simulink model "MIL4L3_SW6_V1_20220211"  (R2018b)
settings: Solver=FixedStepAuto  StartTime=0.0  StopTime=inf  FixedStep=0.001  RelTol=1e-3
PreLoadFcn:
  | A0_MILtest;
undefined symbols (not defined in the file or in its folder): Clb_ICADirect_LaneDisp_StateFive, Clb_ICADirect_LaneDisp_StateFour, Clb_ICADirect_LaneDisp_StateOne, Clb_ICADirect_LaneDisp_StateThree, Clb_ICADirect_LaneDisp_StateTwo, Clb_ICADirect_LaneDisp_StateZero, Clb_ICADirect_LaneDispSW, Clb_ICADirect_TrnLghtsCom_Switch, Clb_ICADirect_TrnLghtsCom_Value, Clb_ICADirect_TrnLghtsCrtl_Inhb, IMAP_Clb_ACU_Driver_Belt, IMAP_Clb_ACU_Driver_Belt_Over, IMAP_Clb_ACU_Passenger_Belt, IMAP_Clb_ACU_Passenger_Belt_Over, IMAP_Clb_ACU_RearLeft_Belt, IMAP_Clb_ACU_RearLeft_Belt_Over, IMAP_Clb_ACU_RearMiddle_Belt, IMAP_Clb_ACU_RearMiddle_Belt_Over, IMAP_Clb_ACU_RearRight_Belt, IMAP_Clb_ACU_RearRight_Belt_Over, IMAP_Clb_AEB_Switch, IMAP_Clb_AEB_Switch_Over, IMAP_Clb_ALC_TLC_Mode, IMAP_Clb_ALC_TLC_Mode_Over, IMAP_Clb_BCM_Battery_Voltage, IMAP_Clb_BCM_Battery_Voltage_Over, IMAP_Clb_BCM_BrakeLamp_State, IMAP_Clb_BCM_BrakeLamp_State_Over, IMAP_Clb_BCM_CHMSL_Status, IMAP_Clb_BCM_CHMSL_Status_Over, IMAP_Clb_BCM_Door_Lock_State, IMAP_Clb_BCM_Door_Lock_State_Over, IMAP_Clb_BCM_FrontWiper_State, IMAP_Clb_BCM_FrontWiper_State_Over, IMAP_Clb_BCM_FrontWiper_Switch, IMAP_Clb_BCM_FrontWiper_Switch_Over, IMAP_Clb_BCM_HazardLamp, IMAP_Clb_BCM_HazardLamp_Over, IMAP_Clb_BCM_HazardLamp_Switch, IMAP_Clb_BCM_HazardLamp_Switch_Over, IMAP_Clb_BCM_HighBeam_State, IMAP_Clb_BCM_HighBeam_State_Over, IMAP_Clb_BCM_Ignition_State, IMAP_Clb_BCM_Ignition_State_Over, IMAP_Clb_BCM_IHBC_Enabled, IMAP_Clb_BCM_IHBC_Enabled_Over, IMAP_Clb_BCM_Left_Light, IMAP_Clb_BCM_Left_Light_Over, IMAP_Clb_BCM_LeftTurn_Switch, IMAP_Clb_BCM_LeftTurn_Switch_Over, IMAP_Clb_BCM_LF_Door_State, IMAP_Clb_BCM_LF_Door_State_Over, IMAP_Clb_BCM_LowBeam_State, IMAP_Clb_BCM_LowBeam_State_Over, IMAP_Clb_BCM_LR_Door_State, IMAP_Clb_BCM_LR_Door_State_Over, IMAP_Clb_BCM_RF_Door_State, IMAP_Clb_BCM_RF_Door_State_Over, IMAP_Clb_BCM_Right_Light, IMAP_Clb_BCM_Right_Light_Over ... (+547)
libraries: CarMaker4SL x2153, simulink x292, dspstat3 x3, canmsglib x2, simulink_extras x1
(part 25 of 52)

== system MIL4L3_SW6_V1_20220211/CarMaker/VehicleControl/Data Inport/SDFA-L3/Subsystem58 ==
  BusCreator : BusCreator  Inputs=10
  Data Type Conversion{1..3,92} (4 alike) : DataTypeConversion  OutDataTypeStr=single
  Ground{,1..5} (6 alike) : Ground
  Read CM Dict1 : CarMaker4SL/Read CM Dict  xname=User.IO.Out.ReferencePoint_S2_002  xsync=off
  Read CM Dict2 : CarMaker4SL/Read CM Dict  xname=User.IO.Out.ReferencePoint_S2_003  xsync=off
  Read CM Dict3 : CarMaker4SL/Read CM Dict  xname=User.IO.Out.ReferencePoint_S2_004  xsync=off
  Read CM Dict5 : CarMaker4SL/Read CM Dict  xname=User.IO.Out.ReferencePoint_S2_001  xsync=off
  LFtar_ReferencePoint : Outport
  wires:
  Data Type Conversion92/1 -> BusCreator/1
  Data Type Conversion3/1 -> BusCreator/4
  Data Type Conversion2/1 -> BusCreator/3
  Data Type Conversion1/1 -> BusCreator/2
  Ground5/1 -> BusCreator/10
  Ground4/1 -> BusCreator/9
  Ground3/1 -> BusCreator/8
  Ground2/1 -> BusCreator/7
  Ground1/1 -> BusCreator/6
  Ground/1 -> BusCreator/5
  Read CM Dict5/1 -> Data Type Conversion92/1
  Read CM Dict1/1 -> Data Type Conversion1/1
  Read CM Dict2/1 -> Data Type Conversion2/1
  Read CM Dict3/1 -> Data Type Conversion3/1
  BusCreator/1 -> LFtar_ReferencePoint/1

== system MIL4L3_SW6_V1_20220211/CarMaker/VehicleControl/Data Inport/SDFA-L3/Subsystem59 ==
  BusCreator : BusCreator  Inputs=10
  Data Type Conversion{1..3,92} (4 alike) : DataTypeConversion  OutDataTypeStr=single
  Ground{,1..5} (6 alike) : Ground
  Read CM Dict1 : CarMaker4SL/Read CM Dict  xname=User.IO.Out.MovingState_S2_002  xsync=off
  Read CM Dict2 : CarMaker4SL/Read CM Dict  xname=User.IO.Out.MovingState_S2_003  xsync=off
  Read CM Dict3 : CarMaker4SL/Read CM Dict  xname=User.IO.Out.MovingState_S2_004  xsync=off
  Read CM Dict5 : CarMaker4SL/Read CM Dict  xname=User.IO.Out.MovingState_S2_001  xsync=off
  LFtar_MovingState : Outport
  wires:
  Data Type Conversion92/1 -> BusCreator/1
  Data Type Conversion3/1 -> BusCreator/4
  Data Type Conversion2/1 -> BusCreator/3
  Data Type Conversion1/1 -> BusCreator/2
  BusCreator/1 -> LFtar_MovingState/1
  Read CM Dict3/1 -> Data Type Conversion3/1
  Read CM Dict2/1 -> Data Type Conversion2/1
  Read CM Dict1/1 -> Data Type Conversion1/1
  Read CM Dict5/1 -> Data Type Conversion92/1
  Ground/1 -> BusCreator/5
  Ground1/1 -> BusCreator/6
  Ground2/1 -> BusCreator/7
  Ground3/1 -> BusCreator/8
  Ground4/1 -> BusCreator/9
  Ground5/1 -> BusCreator/10

== system MIL4L3_SW6_V1_20220211/CarMaker/VehicleControl/Data Inport/SDFA-L3/Subsystem6 ==
  Bus Creator : BusCreator  Inputs=20
  Ground{,1..15} (16 alike) : Ground
  Read CM Dict1 : CarMaker4SL/Read CM Dict  xname=User.IO.Out.IFC_obj02_HeadOrientation  xsync=off
  Read CM Dict2 : CarMaker4SL/Read CM Dict  xname=User.IO.Out.IFC_obj03_HeadOrientation  xsync=off
  Read CM Dict3 : CarMaker4SL/Read CM Dict  xname=User.IO.Out.IFC_obj04_HeadOrientation  xsync=off
  Read CM Dict4 : CarMaker4SL/Read CM Dict  xname=User.IO.Out.IFC_obj01_HeadOrientation  xsync=off
  obj_HeadOrientation : Outport
  wires:
  Bus Creator/1 -> obj_HeadOrientation/1
  Ground15/1 -> Bus Creator/20
  Ground11/1 -> Bus Creator/16
  Ground14/1 -> Bus Creator/19
  Ground12/1 -> Bus Creator/17
  Ground3/1 -> Bus Creator/8
  Ground1/1 -> Bus Creator/6
  Read CM Dict1/1 -> Bus Creator/2
  Read CM Dict4/1 -> Bus Creator/1
  Ground6/1 -> Bus Creator/11
  Ground10/1 -> Bus Creator/15
  Ground13/1 -> Bus Creator/18
  Ground2/1 -> Bus Creator/7
  Ground/1 -> Bus Creator/5
  Ground7/1 -> Bus Creator/12
  Read CM Dict3/1 -> Bus Creator/4
  Ground4/1 -> Bus Creator/9
  Ground9/1 -> Bus Creator/14
  Ground5/1 -> Bus Creator/10
  Ground8/1 -> Bus Creator/13
  Read CM Dict2/1 -> Bus Creator/3

== system MIL4L3_SW6_V1_20220211/CarMaker/VehicleControl/Data Inport/SDFA-L3/Subsystem61 ==
  BusCreator : BusCreator  Inputs=10
  Data Type Conversion{1..3,92} (4 alike) : DataTypeConversion  OutDataTypeStr=single
  Ground{,1..5} (6 alike) : Ground
  Read CM Dict1 : CarMaker4SL/Read CM Dict  xname=User.IO.Out.ClassHighestProb_S2_002  xsync=off
  Read CM Dict2 : CarMaker4SL/Read CM Dict  xname=User.IO.Out.ClassHighestProb_S2_003  xsync=off
  Read CM Dict3 : CarMaker4SL/Read CM Dict  xname=User.IO.Out.ClassHighestProb_S2_004  xsync=off
  Read CM Dict5 : CarMaker4SL/Read CM Dict  xname=User.IO.Out.ClassHighestProb_S2_001  xsync=off
  LFtar_ClassHighestProb : Outport
  wires:
  Data Type Conversion3/1 -> BusCreator/4
  Data Type Conversion92/1 -> BusCreator/1
  Data Type Conversion2/1 -> BusCreator/3
  Data Type Conversion1/1 -> BusCreator/2
  BusCreator/1 -> LFtar_ClassHighestProb/1
  Read CM Dict3/1 -> Data Type Conversion3/1
  Read CM Dict2/1 -> Data Type Conversion2/1
  Read CM Dict1/1 -> Data Type Conversion1/1
  Read CM Dict5/1 -> Data Type Conversion92/1
  Ground/1 -> BusCreator/5
  Ground1/1 -> BusCreator/6
  Ground2/1 -> BusCreator/7
  Ground3/1 -> BusCreator/8
  Ground4/1 -> BusCreator/9
  Ground5/1 -> BusCreator/10

== system MIL4L3_SW6_V1_20220211/CarMaker/VehicleControl/Data Inport/SDFA-L3/Subsystem66 ==
  BusCreator : BusCreator  Inputs=10
  Data Type Conversion{1..3,92} (4 alike) : DataTypeConversion  OutDataTypeStr=uint16
  Ground{,1..5} (6 alike) : Ground
  Read CM Dict1 : CarMaker4SL/Read CM Dict  xname=User.IO.Out.Id_S3_002  xsync=off
  Read CM Dict2 : CarMaker4SL/Read CM Dict  xname=User.IO.Out.Id_S3_003  xsync=off
  Read CM Dict3 : CarMaker4SL/Read CM Dict  xname=User.IO.Out.Id_S3_004  xsync=off
  Read CM Dict5 : CarMaker4SL/Read CM Dict  xname=User.IO.Out.Id_S3_001  xsync=off
  RFtar_id : Outport
  wires:
  Data Type Conversion92/1 -> BusCreator/1
  Data Type Conversion3/1 -> BusCreator/4
  Data Type Conversion2/1 -> BusCreator/3
  Data Type Conversion1/1 -> BusCreator/2
  BusCreator/1 -> RFtar_id/1
  Read CM Dict3/1 -> Data Type Conversion3/1
  Read CM Dict2/1 -> Data Type Conversion2/1
  Read CM Dict1/1 -> Data Type Conversion1/1
  Read CM Dict5/1 -> Data Type Conversion92/1
  Ground/1 -> BusCreator/5
  Ground1/1 -> BusCreator/6
  Ground2/1 -> BusCreator/7
  Ground3/1 -> BusCreator/8
  Ground4/1 -> BusCreator/9
  Ground5/1 -> BusCreator/10

== system MIL4L3_SW6_V1_20220211/CarMaker/VehicleControl/Data Inport/SDFA-L3/Subsystem67 ==
  BusCreator : BusCreator  Inputs=10
  Data Type Conversion{1..3,92} (4 alike) : DataTypeConversion  OutDataTypeStr=single
  Ground{,1..5} (6 alike) : Ground
  Read CM Dict1 : CarMaker4SL/Read CM Dict  xname=User.IO.Out.XPos_S3_002  xsync=off
  Read CM Dict2 : CarMaker4SL/Read CM Dict  xname=User.IO.Out.XPos_S3_003  xsync=off
  Read CM Dict3 : CarMaker4SL/Read CM Dict  xname=User.IO.Out.XPos_S3_004  xsync=off
  Read CM Dict5 : CarMaker4SL/Read CM Dict  xname=User.IO.Out.XPos_S3_001  xsync=off
  RFtar_Xpos : Outport
  wires:
  Data Type Conversion3/1 -> BusCreator/4
  Data Type Conversion92/1 -> BusCreator/1
  Data Type Conversion2/1 -> BusCreator/3
  Data Type Conversion1/1 -> BusCreator/2
  Ground5/1 -> BusCreator/10
  Ground4/1 -> BusCreator/9
  Ground3/1 -> BusCreator/8
  Ground2/1 -> BusCreator/7
  Ground1/1 -> BusCreator/6
  Ground/1 -> BusCreator/5
  Read CM Dict5/1 -> Data Type Conversion92/1
  Read CM Dict1/1 -> Data Type Conversion1/1
  Read CM Dict2/1 -> Data Type Conversion2/1
  Read CM Dict3/1 -> Data Type Conversion3/1
  BusCreator/1 -> RFtar_Xpos/1

== system MIL4L3_SW6_V1_20220211/CarMaker/VehicleControl/Data Inport/SDFA-L3/Subsystem68 ==
  BusCreator : BusCreator  Inputs=10
  Data Type Conversion{1..3,92} (4 alike) : DataTypeConversion  OutDataTypeStr=single
  Ground{,1..5} (6 alike) : Ground
  Read CM Dict1 : CarMaker4SL/Read CM Dict  xname=User.IO.Out.YPos_S3_002  xsync=off
  Read CM Dict2 : CarMaker4SL/Read CM Dict  xname=User.IO.Out.YPos_S3_003  xsync=off
  Read CM Dict3 : CarMaker4SL/Read CM Dict  xname=User.IO.Out.YPos_S3_004  xsync=off
  Read CM Dict5 : CarMaker4SL/Read CM Dict  xname=User.IO.Out.YPos_S3_001  xsync=off
  RFtar_Ypos : Outport
  wires:
  Data Type Conversion92/1 -> BusCreator/1
  Data Type Conversion2/1 -> BusCreator/3
  Data Type Conversion3/1 -> BusCreator/4
  Data Type Conversion1/1 -> BusCreator/2
  BusCreator/1 -> RFtar_Ypos/1
  Read CM Dict3/1 -> Data Type Conversion3/1
  Read CM Dict2/1 -> Data Type Conversion2/1
  Read CM Dict1/1 -> Data Type Conversion1/1
  Read CM Dict5/1 -> Data Type Conversion92/1
  Ground/1 -> BusCreator/5
  Ground1/1 -> BusCreator/6
  Ground2/1 -> BusCreator/7
  Ground3/1 -> BusCreator/8
  Ground4/1 -> BusCreator/9
  Ground5/1 -> BusCreator/10

== system MIL4L3_SW6_V1_20220211/CarMaker/VehicleControl/Data Inport/SDFA-L3/Subsystem69 ==
  BusCreator : BusCreator  Inputs=10
  Data Type Conversion{1..3,92} (4 alike) : DataTypeConversion  OutDataTypeStr=single
  Ground{,1..5} (6 alike) : Ground
  Read CM Dict1 : CarMaker4SL/Read CM Dict  xname=User.IO.Out.XVelocity_S3_002  xsync=off
  Read CM Dict2 : CarMaker4SL/Read CM Dict  xname=User.IO.Out.XVelocity_S3_003  xsync=off
  Read CM Dict3 : CarMaker4SL/Read CM Dict  xname=User.IO.Out.XVelocity_S3_004  xsync=off
  Read CM Dict5 : CarMaker4SL/Read CM Dict  xname=User.IO.Out.XVelocity_S3_001  xsync=off
  RFtar_Xvelocity : Outport
  wires:
  Data Type Conversion2/1 -> BusCreator/3
  Data Type Conversion1/1 -> BusCreator/2
  Data Type Conversion92/1 -> BusCreator/1
  Data Type Conversion3/1 -> BusCreator/4
  Ground5/1 -> BusCreator/10
  Ground4/1 -> BusCreator/9
  Ground3/1 -> BusCreator/8
  Ground2/1 -> BusCreator/7
  Ground1/1 -> BusCreator/6
  Ground/1 -> BusCreator/5
  Read CM Dict5/1 -> Data Type Conversion92/1
  Read CM Dict1/1 -> Data Type Conversion1/1
  Read CM Dict2/1 -> Data Type Conversion2/1
  Read CM Dict3/1 -> Data Type Conversion3/1
  BusCreator/1 -> RFtar_Xvelocity/1

== system MIL4L3_SW6_V1_20220211/CarMaker/VehicleControl/Data Inport/SDFA-L3/Subsystem7 ==
  Bus Creator : BusCreator  Inputs=20
  Ground{,1..15} (16 alike) : Ground
  Read CM Dict : CarMaker4SL/Read CM Dict  xname=User.IO.Out.IFC_obj01_DirIndicator  xsync=off
  Read CM Dict1 : CarMaker4SL/Read CM Dict  xname=User.IO.Out.IFC_obj02_DirIndicator  xsync=off
  Read CM Dict2 : CarMaker4SL/Read CM Dict  xname=User.IO.Out.IFC_obj03_DirIndicator  xsync=off
  Read CM Dict3 : CarMaker4SL/Read CM Dict  xname=User.IO.Out.IFC_obj04_DirIndicator  xsync=off
  obj_DirIndicator : Outport
  wires:
  Read CM Dict2/1 -> Bus Creator/3
  Ground8/1 -> Bus Creator/13
  Ground5/1 -> Bus Creator/10
  Ground9/1 -> Bus Creator/14
  Ground4/1 -> Bus Creator/9
  Read CM Dict3/1 -> Bus Creator/4
  Ground7/1 -> Bus Creator/12
  Ground/1 -> Bus Creator/5
  Ground2/1 -> Bus Creator/7
  Ground13/1 -> Bus Creator/18
  Ground10/1 -> Bus Creator/15
  Ground6/1 -> Bus Creator/11
  Read CM Dict/1 -> Bus Creator/1
  Read CM Dict1/1 -> Bus Creator/2
  Ground1/1 -> Bus Creator/6
  Ground3/1 -> Bus Creator/8
  Ground12/1 -> Bus Creator/17
  Ground14/1 -> Bus Creator/19
  Ground11/1 -> Bus Creator/16
  Ground15/1 -> Bus Creator/20
  Bus Creator/1 -> obj_DirIndicator/1

== system MIL4L3_SW6_V1_20220211/CarMaker/VehicleControl/Data Inport/SDFA-L3/Subsystem70 ==
  BusCreator : BusCreator  Inputs=10
  Data Type Conversion{1..3,92} (4 alike) : DataTypeConversion  OutDataTypeStr=single
  Ground{,1..5} (6 alike) : Ground
  Read CM Dict1 : CarMaker4SL/Read CM Dict  xname=User.IO.Out.YVelocity_S3_002  xsync=off
  Read CM Dict2 : CarMaker4SL/Read CM Dict  xname=User.IO.Out.YVelocity_S3_003  xsync=off
  Read CM Dict3 : CarMaker4SL/Read CM Dict  xname=User.IO.Out.YVelocity_S3_004  xsync=off
  Read CM Dict5 : CarMaker4SL/Read CM Dict  xname=User.IO.Out.YVelocity_S3_001  xsync=off
  RFtar_Yvelocity : Outport
  wires:
  Data Type Conversion92/1 -> BusCreator/1
  Data Type Conversion2/1 -> BusCreator/3
  Data Type Conversion3/1 -> BusCreator/4
  Data Type Conversion1/1 -> BusCreator/2
  BusCreator/1 -> RFtar_Yvelocity/1
  Read CM Dict3/1 -> Data Type Conversion3/1
  Read CM Dict2/1 -> Data Type Conversion2/1
  Read CM Dict1/1 -> Data Type Conversion1/1
  Read CM Dict5/1 -> Data Type Conversion92/1
  Ground/1 -> BusCreator/5
  Ground1/1 -> BusCreator/6
  Ground2/1 -> BusCreator/7
  Ground3/1 -> BusCreator/8
  Ground4/1 -> BusCreator/9
  Ground5/1 -> BusCreator/10

== system MIL4L3_SW6_V1_20220211/CarMaker/VehicleControl/Data Inport/SDFA-L3/Subsystem71 ==
  BusCreator : BusCreator  Inputs=10
  Data Type Conversion{1..3,92} (4 alike) : DataTypeConversion  OutDataTypeStr=single
  Ground{,1..5} (6 alike) : Ground
  Read CM Dict1 : CarMaker4SL/Read CM Dict  xname=User.IO.Out.XAcceleration_S3_002  xsync=off
  Read CM Dict2 : CarMaker4SL/Read CM Dict  xname=User.IO.Out.XAcceleration_S3_003  xsync=off
  Read CM Dict3 : CarMaker4SL/Read CM Dict  xname=User.IO.Out.XAcceleration_S3_004  xsync=off
  Read CM Dict5 : CarMaker4SL/Read CM Dict  xname=User.IO.Out.XAcceleration_S3_001  xsync=off
  RFtar_Xacceleration : Outport
  wires:
  Data Type Conversion92/1 -> BusCreator/1
  Data Type Conversion3/1 -> BusCreator/4
  Data Type Conversion1/1 -> BusCreator/2
  Data Type Conversion2/1 -> BusCreator/3
  Ground5/1 -> BusCreator/10
  Ground4/1 -> BusCreator/9
  Ground3/1 -> BusCreator/8
  Ground2/1 -> BusCreator/7
  Ground1/1 -> BusCreator/6
  Ground/1 -> BusCreator/5
  Read CM Dict5/1 -> Data Type Conversion92/1
  Read CM Dict1/1 -> Data Type Conversion1/1
  Read CM Dict2/1 -> Data Type Conversion2/1
  Read CM Dict3/1 -> Data Type Conversion3/1
  BusCreator/1 -> RFtar_Xacceleration/1

== system MIL4L3_SW6_V1_20220211/CarMaker/VehicleControl/Data Inport/SDFA-L3/Subsystem72 ==
  BusCreator : BusCreator  Inputs=10
  Data Type Conversion{1..3,92} (4 alike) : DataTypeConversion  OutDataTypeStr=single
  Ground{,1..5} (6 alike) : Ground
  Read CM Dict1 : CarMaker4SL/Read CM Dict  xname=User.IO.Out.YAcceleration_S3_002  xsync=off
  Read CM Dict2 : CarMaker4SL/Read CM Dict  xname=User.IO.Out.YAcceleration_S3_003  xsync=off
  Read CM Dict3 : CarMaker4SL/Read CM Dict  xname=User.IO.Out.YAcceleration_S3_004  xsync=off
  Read CM Dict5 : CarMaker4SL/Read CM Dict  xname=User.IO.Out.YAcceleration_S3_001  xsync=off
  RFtar_Yacceleration : Outport
  wires:
  Data Type Conversion92/1 -> BusCreator/1
  Data Type Conversion3/1 -> BusCreator/4
  Data Type Conversion2/1 -> BusCreator/3
  Data Type Conversion1/1 -> BusCreator/2
  BusCreator/1 -> RFtar_Yacceleration/1
  Read CM Dict3/1 -> Data Type Conversion3/1
  Read CM Dict2/1 -> Data Type Conversion2/1
  Read CM Dict1/1 -> Data Type Conversion1/1
  Read CM Dict5/1 -> Data Type Conversion92/1
  Ground/1 -> BusCreator/5
  Ground1/1 -> BusCreator/6
  Ground2/1 -> BusCreator/7
  Ground3/1 -> BusCreator/8
  Ground4/1 -> BusCreator/9
  Ground5/1 -> BusCreator/10

== system MIL4L3_SW6_V1_20220211/CarMaker/VehicleControl/Data Inport/SDFA-L3/Subsystem73 ==
  BusCreator : BusCreator  Inputs=10
  Data Type Conversion{1..3,92} (4 alike) : DataTypeConversion  OutDataTypeStr=single
  Ground{,1..5} (6 alike) : Ground
  Read CM Dict1 : CarMaker4SL/Read CM Dict  xname=User.IO.Out.Width_S3_002  xsync=off
  Read CM Dict2 : CarMaker4SL/Read CM Dict  xname=User.IO.Out.Width_S3_003  xsync=off
  Read CM Dict3 : CarMaker4SL/Read CM Dict  xname=User.IO.Out.Width_S3_004  xsync=off
  Read CM Dict5 : CarMaker4SL/Read CM Dict  xname=User.IO.Out.Width_S3_001  xsync=off
  RFtar_Width : Outport
  wires:
  Data Type Conversion92/1 -> BusCreator/1
  Data Type Conversion2/1 -> BusCreator/3
  Data Type Conversion1/1 -> BusCreator/2
  Data Type Conversion3/1 -> BusCreator/4
  Ground5/1 -> BusCreator/10
  Ground4/1 -> BusCreator/9
  Ground3/1 -> BusCreator/8
  Ground2/1 -> BusCreator/7
  Ground1/1 -> BusCreator/6
  Ground/1 -> BusCreator/5
  Read CM Dict5/1 -> Data Type Conversion92/1
  Read CM Dict1/1 -> Data Type Conversion1/1
  Read CM Dict2/1 -> Data Type Conversion2/1
  Read CM Dict3/1 -> Data Type Conversion3/1
  BusCreator/1 -> RFtar_Width/1

== system MIL4L3_SW6_V1_20220211/CarMaker/VehicleControl/Data Inport/SDFA-L3/Subsystem74 ==
  BusCreator : BusCreator  Inputs=10
  Data Type Conversion{1..3,92} (4 alike) : DataTypeConversion  OutDataTypeStr=single
  Ground{,1..5} (6 alike) : Ground
  Read CM Dict1 : CarMaker4SL/Read CM Dict  xname=User.IO.Out.Length_S3_002  xsync=off
  Read CM Dict2 : CarMaker4SL/Read CM Dict  xname=User.IO.Out.Length_S3_003  xsync=off
  Read CM Dict3 : CarMaker4SL/Read CM Dict  xname=User.IO.Out.Length_S3_004  xsync=off
  Read CM Dict5 : CarMaker4SL/Read CM Dict  xname=User.IO.Out.Length_S3_001  xsync=off
  RFtar_Length : Outport
  wires:
  Data Type Conversion2/1 -> BusCreator/3
  Data Type Conversion3/1 -> BusCreator/4
  Data Type Conversion92/1 -> BusCreator/1
  Data Type Conversion1/1 -> BusCreator/2
  BusCreator/1 -> RFtar_Length/1
  Read CM Dict3/1 -> Data Type Conversion3/1
  Read CM Dict2/1 -> Data Type Conversion2/1
  Read CM Dict1/1 -> Data Type Conversion1/1
  Read CM Dict5/1 -> Data Type Conversion92/1
  Ground/1 -> BusCreator/5
  Ground1/1 -> BusCreator/6
  Ground2/1 -> BusCreator/7
  Ground3/1 -> BusCreator/8
  Ground4/1 -> BusCreator/9
  Ground5/1 -> BusCreator/10

== system MIL4L3_SW6_V1_20220211/CarMaker/VehicleControl/Data Inport/SDFA-L3/Subsystem75 ==
  BusCreator : BusCreator  Inputs=10
  Data Type Conversion{1..3,92} (4 alike) : DataTypeConversion  OutDataTypeStr=single
  Ground{,1..5} (6 alike) : Ground
  Read CM Dict1 : CarMaker4SL/Read CM Dict  xname=User.IO.Out.Orientation_S3_002  xsync=off
  Read CM Dict2 : CarMaker4SL/Read CM Dict  xname=User.IO.Out.Orientation_S3_003  xsync=off
  Read CM Dict3 : CarMaker4SL/Read CM Dict  xname=User.IO.Out.Orientation_S3_004  xsync=off
  Read CM Dict5 : CarMaker4SL/Read CM Dict  xname=User.IO.Out.Orientation_S3_001  xsync=off
  RFtar_Orientation : Outport
  wires:
  Data Type Conversion92/1 -> BusCreator/1
  Data Type Conversion2/1 -> BusCreator/3
  Data Type Conversion1/1 -> BusCreator/2
  Data Type Conversion3/1 -> BusCreator/4
  Ground5/1 -> BusCreator/10
  Ground4/1 -> BusCreator/9
  Ground3/1 -> BusCreator/8
  Ground2/1 -> BusCreator/7
  Ground1/1 -> BusCreator/6
  Ground/1 -> BusCreator/5
  Read CM Dict5/1 -> Data Type Conversion92/1
  Read CM Dict1/1 -> Data Type Conversion1/1
  Read CM Dict2/1 -> Data Type Conversion2/1
  Read CM Dict3/1 -> Data Type Conversion3/1
  BusCreator/1 -> RFtar_Orientation/1

== system MIL4L3_SW6_V1_20220211/CarMaker/VehicleControl/Data Inport/SDFA-L3/Subsystem76 ==
  BusCreator : BusCreator  Inputs=10
  Data Type Conversion{1..3,92} (4 alike) : DataTypeConversion  OutDataTypeStr=single
  Ground{,1..5} (6 alike) : Ground
  Read CM Dict1 : CarMaker4SL/Read CM Dict  xname=User.IO.Out.ExistenceProbability_S3_002  xsync=off
  Read CM Dict2 : CarMaker4SL/Read CM Dict  xname=User.IO.Out.ExistenceProbability_S3_003  xsync=off
  Read CM Dict3 : CarMaker4SL/Read CM Dict  xname=User.IO.Out.ExistenceProbability_S3_004  xsync=off
  Read CM Dict5 : CarMaker4SL/Read CM Dict  xname=User.IO.Out.ExistenceProbability_S3_001  xsync=off
  RFtar_ExistenceProbability : Outport
  wires:
  Data Type Conversion2/1 -> BusCreator/3
  Data Type Conversion3/1 -> BusCreator/4
  Data Type Conversion1/1 -> BusCreator/2
  Data Type Conversion92/1 -> BusCreator/1
  BusCreator/1 -> RFtar_ExistenceProbability/1
  Read CM Dict3/1 -> Data Type Conversion3/1
  Read CM Dict2/1 -> Data Type Conversion2/1
  Read CM Dict1/1 -> Data Type Conversion1/1
  Read CM Dict5/1 -> Data Type Conversion92/1
  Ground/1 -> BusCreator/5
  Ground1/1 -> BusCreator/6
  Ground2/1 -> BusCreator/7
  Ground3/1 -> BusCreator/8
  Ground4/1 -> BusCreator/9
  Ground5/1 -> BusCreator/10

== system MIL4L3_SW6_V1_20220211/CarMaker/VehicleControl/Data Inport/SDFA-L3/Subsystem77 ==
  BusCreator : BusCreator  Inputs=10
  Data Type Conversion{1..3,92} (4 alike) : DataTypeConversion  OutDataTypeStr=uint8
  Ground{,1..5} (6 alike) : Ground
  Read CM Dict1 : CarMaker4SL/Read CM Dict  xname=User.IO.Out.ClassHighest_S3_002  xsync=off
  Read CM Dict2 : CarMaker4SL/Read CM Dict  xname=User.IO.Out.ClassHighest_S3_003  xsync=off
  Read CM Dict3 : CarMaker4SL/Read CM Dict  xname=User.IO.Out.ClassHighest_S3_004  xsync=off
  Read CM Dict5 : CarMaker4SL/Read CM Dict  xname=User.IO.Out.ClassHighest_S3_001  xsync=off
  RFtar_Class : Outport
  wires:
  Data Type Conversion3/1 -> BusCreator/4
  Data Type Conversion2/1 -> BusCreator/3
  Data Type Conversion92/1 -> BusCreator/1
  Data Type Conversion1/1 -> BusCreator/2
  Ground5/1 -> BusCreator/10
  Ground4/1 -> BusCreator/9
  Ground3/1 -> BusCreator/8
  Ground2/1 -> BusCreator/7
  Ground1/1 -> BusCreator/6
  Ground/1 -> BusCreator/5
  Read CM Dict5/1 -> Data Type Conversion92/1
  Read CM Dict1/1 -> Data Type Conversion1/1
  Read CM Dict2/1 -> Data Type Conversion2/1
  Read CM Dict3/1 -> Data Type Conversion3/1
  BusCreator/1 -> RFtar_Class/1

== system MIL4L3_SW6_V1_20220211/CarMaker/VehicleControl/Data Inport/SDFA-L3/Subsystem78 ==
  BusCreator : BusCreator  Inputs=10
  Data Type Conversion{1..3,92} (4 alike) : DataTypeConversion  OutDataTypeStr=single
  Ground{,1..5} (6 alike) : Ground
  Read CM Dict1 : CarMaker4SL/Read CM Dict  xname=User.IO.Out.ReferencePoint_S3_002  xsync=off
  Read CM Dict2 : CarMaker4SL/Read CM Dict  xname=User.IO.Out.ReferencePoint_S3_003  xsync=off
  Read CM Dict3 : CarMaker4SL/Read CM Dict  xname=User.IO.Out.ReferencePoint_S3_004  xsync=off
  Read CM Dict5 : CarMaker4SL/Read CM Dict  xname=User.IO.Out.ReferencePoint_S3_001  xsync=off
  RFtar_ReferencePoint : Outport
  wires:
  Data Type Conversion1/1 -> BusCreator/2
  Data Type Conversion3/1 -> BusCreator/4
  Data Type Conversion2/1 -> BusCreator/3
  Data Type Conversion92/1 -> BusCreator/1
  BusCreator/1 -> RFtar_ReferencePoint/1
  Read CM Dict3/1 -> Data Type Conversion3/1
  Read CM Dict2/1 -> Data Type Conversion2/1
  Read CM Dict1/1 -> Data Type Conversion1/1
  Read CM Dict5/1 -> Data Type Conversion92/1
  Ground/1 -> BusCreator/5
  Ground1/1 -> BusCreator/6
  Ground2/1 -> BusCreator/7
  Ground3/1 -> BusCreator/8
  Ground4/1 -> BusCreator/9
  Ground5/1 -> BusCreator/10

== system MIL4L3_SW6_V1_20220211/CarMaker/VehicleControl/Data Inport/SDFA-L3/Subsystem79 ==
  BusCreator : BusCreator  Inputs=10
  Data Type Conversion{1..3,92} (4 alike) : DataTypeConversion  OutDataTypeStr=single
  Ground{,1..5} (6 alike) : Ground
  Read CM Dict1 : CarMaker4SL/Read CM Dict  xname=User.IO.Out.MovingState_S3_002  xsync=off
  Read CM Dict2 : CarMaker4SL/Read CM Dict  xname=User.IO.Out.MovingState_S3_003  xsync=off
  Read CM Dict3 : CarMaker4SL/Read CM Dict  xname=User.IO.Out.MovingState_S3_004  xsync=off
  Read CM Dict5 : CarMaker4SL/Read CM Dict  xname=User.IO.Out.MovingState_S3_001  xsync=off
  RFtar_MovingState : Outport
  wires:
  Data Type Conversion3/1 -> BusCreator/4
  Data Type Conversion92/1 -> BusCreator/1
  Data Type Conversion2/1 -> BusCreator/3
  Data Type Conversion1/1 -> BusCreator/2
  Ground5/1 -> BusCreator/10
  Ground4/1 -> BusCreator/9
  Ground3/1 -> BusCreator/8
  Ground2/1 -> BusCreator/7
  Ground1/1 -> BusCreator/6
  Ground/1 -> BusCreator/5
  Read CM Dict5/1 -> Data Type Conversion92/1
  Read CM Dict1/1 -> Data Type Conversion1/1
  Read CM Dict2/1 -> Data Type Conversion2/1
  Read CM Dict3/1 -> Data Type Conversion3/1
  BusCreator/1 -> RFtar_MovingState/1

== system MIL4L3_SW6_V1_20220211/CarMaker/VehicleControl/Data Inport/SDFA-L3/Subsystem8 ==
  Bus Creator : BusCreator  Inputs=20
  Ground{,1..15} (16 alike) : Ground
  Read CM Dict : CarMaker4SL/Read CM Dict  xname=User.IO.Out.IFC_obj01_angle_rate  xsync=off
  Read CM Dict1 : CarMaker4SL/Read CM Dict  xname=User.IO.Out.IFC_obj02_angle_rate  xsync=off
  Read CM Dict2 : CarMaker4SL/Read CM Dict  xname=User.IO.Out.IFC_obj03_angle_rate  xsync=off
  Read CM Dict3 : CarMaker4SL/Read CM Dict  xname=User.IO.Out.IFC_obj04_angle_rate  xsync=off
  obj_angle_rate : Outport
  wires:
  Read CM Dict2/1 -> Bus Creator/3
  Ground8/1 -> Bus Creator/13
  Ground5/1 -> Bus Creator/10
  Ground9/1 -> Bus Creator/14
  Ground4/1 -> Bus Creator/9
  Read CM Dict3/1 -> Bus Creator/4
  Ground7/1 -> Bus Creator/12
  Ground/1 -> Bus Creator/5
  Ground2/1 -> Bus Creator/7
  Ground13/1 -> Bus Creator/18
  Ground10/1 -> Bus Creator/15
  Ground6/1 -> Bus Creator/11
  Read CM Dict/1 -> Bus Creator/1
  Read CM Dict1/1 -> Bus Creator/2
  Ground1/1 -> Bus Creator/6
  Ground3/1 -> Bus Creator/8
  Ground12/1 -> Bus Creator/17
  Ground14/1 -> Bus Creator/19
  Ground11/1 -> Bus Creator/16
  Ground15/1 -> Bus Creator/20
  Bus Creator/1 -> obj_angle_rate/1

== system MIL4L3_SW6_V1_20220211/CarMaker/VehicleControl/Data Inport/SDFA-L3/Subsystem81 ==
  BusCreator : BusCreator  Inputs=10
  Data Type Conversion{1..3,92} (4 alike) : DataTypeConversion  OutDataTypeStr=single
  Ground{,1..5} (6 alike) : Ground
  Read CM Dict1 : CarMaker4SL/Read CM Dict  xname=User.IO.Out.ClassHighestProb_S3_002  xsync=off
  Read CM Dict2 : CarMaker4SL/Read CM Dict  xname=User.IO.Out.ClassHighestProb_S3_003  xsync=off
  Read CM Dict3 : CarMaker4SL/Read CM Dict  xname=User.IO.Out.ClassHighestProb_S3_004  xsync=off
  Read CM Dict5 : CarMaker4SL/Read CM Dict  xname=User.IO.Out.ClassHighestProb_S3_001  xsync=off
  RFtar_ClassHighestProb : Outport
  wires:
  Data Type Conversion92/1 -> BusCreator/1
  Data Type Conversion2/1 -> BusCreator/3
  Data Type Conversion3/1 -> BusCreator/4
  Data Type Conversion1/1 -> BusCreator/2
  Ground5/1 -> BusCreator/10
  Ground4/1 -> BusCreator/9
  Ground3/1 -> BusCreator/8
  Ground2/1 -> BusCreator/7
  Ground1/1 -> BusCreator/6
  Ground/1 -> BusCreator/5
  Read CM Dict5/1 -> Data Type Conversion92/1
  Read CM Dict1/1 -> Data Type Conversion1/1
  Read CM Dict2/1 -> Data Type Conversion2/1
  Read CM Dict3/1 -> Data Type Conversion3/1
  BusCreator/1 -> RFtar_ClassHighestProb/1

== system MIL4L3_SW6_V1_20220211/CarMaker/VehicleControl/Data Inport/SDFA-L3/Subsystem85 ==
  BusCreator : BusCreator  Inputs=10
  Data Type Conversion{1..3,92} (4 alike) : DataTypeConversion  OutDataTypeStr=uint16
  Ground{,1..5} (6 alike) : Ground
  Read CM Dict1 : CarMaker4SL/Read CM Dict  xname=User.IO.Out.Id_S0_002  xsync=off
  Read CM Dict2 : CarMaker4SL/Read CM Dict  xname=User.IO.Out.Id_S0_003  xsync=off
  Read CM Dict3 : CarMaker4SL/Read CM Dict  xname=User.IO.Out.Id_S0_004  xsync=off
  Read CM Dict5 : CarMaker4SL/Read CM Dict  xname=User.IO.Out.Id_S0_001  xsync=off
  LBtar_id : Outport
  wires:
  Data Type Conversion92/1 -> BusCreator/1
  Data Type Conversion3/1 -> BusCreator/4
  Data Type Conversion2/1 -> BusCreator/3
  Data Type Conversion1/1 -> BusCreator/2
  Ground5/1 -> BusCreator/10
  Ground4/1 -> BusCreator/9
  Ground3/1 -> BusCreator/8
  Ground2/1 -> BusCreator/7
  Ground1/1 -> BusCreator/6
  Ground/1 -> BusCreator/5
  Read CM Dict5/1 -> Data Type Conversion92/1
  Read CM Dict1/1 -> Data Type Conversion1/1
  Read CM Dict2/1 -> Data Type Conversion2/1
  Read CM Dict3/1 -> Data Type Conversion3/1
  BusCreator/1 -> LBtar_id/1

== system MIL4L3_SW6_V1_20220211/CarMaker/VehicleControl/Data Inport/SDFA-L3/Subsystem86 ==
  BusCreator : BusCreator  Inputs=10
  Data Type Conversion{1..3,92} (4 alike) : DataTypeConversion  OutDataTypeStr=single
  Ground{,1..5} (6 alike) : Ground
  Read CM Dict1 : CarMaker4SL/Read CM Dict  xname=User.IO.Out.XPos_S0_002  xsync=off
  Read CM Dict2 : CarMaker4SL/Read CM Dict  xname=User.IO.Out.XPos_S0_003  xsync=off
  Read CM Dict3 : CarMaker4SL/Read CM Dict  xname=User.IO.Out.XPos_S0_004  xsync=off
  Read CM Dict5 : CarMaker4SL/Read CM Dict  xname=User.IO.Out.XPos_S0_001  xsync=off
  LBtar_Xpos : Outport
  wires:
  BusCreator/1 -> LBtar_Xpos/1
  Read CM Dict3/1 -> Data Type Conversion3/1
  Read CM Dict2/1 -> Data Type Conversion2/1
  Read CM Dict1/1 -> Data Type Conversion1/1
  Read CM Dict5/1 -> Data Type Conversion92/1
  Ground/1 -> BusCreator/5
  Ground1/1 -> BusCreator/6
  Ground2/1 -> BusCreator/7
  Ground3/1 -> BusCreator/8
  Ground4/1 -> BusCreator/9
  Ground5/1 -> BusCreator/10
  Data Type Conversion92/1 -> BusCreator/1
  Data Type Conversion1/1 -> BusCreator/2
  Data Type Conversion2/1 -> BusCreator/3
  Data Type Conversion3/1 -> BusCreator/4

== system MIL4L3_SW6_V1_20220211/CarMaker/VehicleControl/Data Inport/SDFA-L3/Subsystem87 ==
  BusCreator : BusCreator  Inputs=10
  Data Type Conversion{1..3,92} (4 alike) : DataTypeConversion  OutDataTypeStr=single
  Ground{,1..5} (6 alike) : Ground
  Read CM Dict1 : CarMaker4SL/Read CM Dict  xname=User.IO.Out.YPos_S0_002  xsync=off
  Read CM Dict2 : CarMaker4SL/Read CM Dict  xname=User.IO.Out.YPos_S0_003  xsync=off
  Read CM Dict3 : CarMaker4SL/Read CM Dict  xname=User.IO.Out.YPos_S0_004  xsync=off
  Read CM Dict5 : CarMaker4SL/Read CM Dict  xname=User.IO.Out.YPos_S0_001  xsync=off
  LBtar_Ypos : Outport
  wires:
  Data Type Conversion2/1 -> BusCreator/3
  Data Type Conversion92/1 -> BusCreator/1
  Data Type Conversion3/1 -> BusCreator/4
  Data Type Conversion1/1 -> BusCreator/2
  Ground5/1 -> BusCreator/10
  Ground4/1 -> BusCreator/9
  Ground3/1 -> BusCreator/8
  Ground2/1 -> BusCreator/7
  Ground1/1 -> BusCreator/6
  Ground/1 -> BusCreator/5
  Read CM Dict5/1 -> Data Type Conversion92/1
  Read CM Dict1/1 -> Data Type Conversion1/1
  Read CM Dict2/1 -> Data Type Conversion2/1
  Read CM Dict3/1 -> Data Type Conversion3/1
  BusCreator/1 -> LBtar_Ypos/1

== system MIL4L3_SW6_V1_20220211/CarMaker/VehicleControl/Data Inport/SDFA-L3/Subsystem88 ==
  BusCreator : BusCreator  Inputs=10
  Data Type Conversion{1..3,92} (4 alike) : DataTypeConversion  OutDataTypeStr=single
  Ground{,1..5} (6 alike) : Ground
  Read CM Dict1 : CarMaker4SL/Read CM Dict  xname=User.IO.Out.XVelocity_S0_002  xsync=off
  Read CM Dict2 : CarMaker4SL/Read CM Dict  xname=User.IO.Out.XVelocity_S0_003  xsync=off
  Read CM Dict3 : CarMaker4SL/Read CM Dict  xname=User.IO.Out.XVelocity_S0_004  xsync=off
  Read CM Dict5 : CarMaker4SL/Read CM Dict  xname=User.IO.Out.XVelocity_S0_001  xsync=off
  LBtar_Xvelocity : Outport
  wires:
  Data Type Conversion92/1 -> BusCreator/1
  Data Type Conversion2/1 -> BusCreator/3
  Data Type Conversion3/1 -> BusCreator/4
  Data Type Conversion1/1 -> BusCreator/2
  BusCreator/1 -> LBtar_Xvelocity/1
  Read CM Dict3/1 -> Data Type Conversion3/1
  Read CM Dict2/1 -> Data Type Conversion2/1
  Read CM Dict1/1 -> Data Type Conversion1/1
  Read CM Dict5/1 -> Data Type Conversion92/1
  Ground/1 -> BusCreator/5
  Ground1/1 -> BusCreator/6
  Ground2/1 -> BusCreator/7
  Ground3/1 -> BusCreator/8
  Ground4/1 -> BusCreator/9
  Ground5/1 -> BusCreator/10

== system MIL4L3_SW6_V1_20220211/CarMaker/VehicleControl/Data Inport/SDFA-L3/Subsystem89 ==
  BusCreator : BusCreator  Inputs=10
  Data Type Conversion{1..3,92} (4 alike) : DataTypeConversion  OutDataTypeStr=single
  Ground{,1..5} (6 alike) : Ground
  Read CM Dict1 : CarMaker4SL/Read CM Dict  xname=User.IO.Out.YVelocity_S0_002  xsync=off
  Read CM Dict2 : CarMaker4SL/Read CM Dict  xname=User.IO.Out.YVelocity_S0_003  xsync=off
  Read CM Dict3 : CarMaker4SL/Read CM Dict  xname=User.IO.Out.YVelocity_S0_004  xsync=off
  Read CM Dict5 : CarMaker4SL/Read CM Dict  xname=User.IO.Out.YVelocity_S0_001  xsync=off
  LBtar_Yvelocity : Outport
  wires:
  Data Type Conversion92/1 -> BusCreator/1
  Data Type Conversion2/1 -> BusCreator/3
  Data Type Conversion3/1 -> BusCreator/4
  Data Type Conversion1/1 -> BusCreator/2
  Ground5/1 -> BusCreator/10
  Ground4/1 -> BusCreator/9
  Ground3/1 -> BusCreator/8
  Ground2/1 -> BusCreator/7
  Ground1/1 -> BusCreator/6
  Ground/1 -> BusCreator/5
  Read CM Dict5/1 -> Data Type Conversion92/1
  Read CM Dict1/1 -> Data Type Conversion1/1
  Read CM Dict2/1 -> Data Type Conversion2/1
  Read CM Dict3/1 -> Data Type Conversion3/1
  BusCreator/1 -> LBtar_Yvelocity/1

== system MIL4L3_SW6_V1_20220211/CarMaker/VehicleControl/Data Inport/SDFA-L3/Subsystem9 ==
  Bus Creator : BusCreator  Inputs=20
  Ground{,1..15} (16 alike) : Ground
  Read CM Dict : CarMaker4SL/Read CM Dict  xname=User.IO.Out.IFC_obj01_angle_3D  xsync=off
  Read CM Dict1 : CarMaker4SL/Read CM Dict  xname=User.IO.Out.IFC_obj02_angle_3D  xsync=off
  Read CM Dict2 : CarMaker4SL/Read CM Dict  xname=User.IO.Out.IFC_obj03_angle_3D  xsync=off
  Read CM Dict3 : CarMaker4SL/Read CM Dict  xname=User.IO.Out.IFC_obj04_angle_3D  xsync=off
  obj_angle_3D : Outport
  wires:
  Bus Creator/1 -> obj_angle_3D/1
  Ground15/1 -> Bus Creator/20
  Ground11/1 -> Bus Creator/16
  Ground14/1 -> Bus Creator/19
  Ground12/1 -> Bus Creator/17
  Ground3/1 -> Bus Creator/8
  Ground1/1 -> Bus Creator/6
  Read CM Dict1/1 -> Bus Creator/2
  Read CM Dict/1 -> Bus Creator/1
  Ground6/1 -> Bus Creator/11
  Ground10/1 -> Bus Creator/15
  Ground13/1 -> Bus Creator/18
  Ground2/1 -> Bus Creator/7
  Ground/1 -> Bus Creator/5
  Ground7/1 -> Bus Creator/12
  Read CM Dict3/1 -> Bus Creator/4
  Ground4/1 -> Bus Creator/9
  Ground9/1 -> Bus Creator/14
  Ground5/1 -> Bus Creator/10
  Ground8/1 -> Bus Creator/13
  Read CM Dict2/1 -> Bus Creator/3

== system MIL4L3_SW6_V1_20220211/CarMaker/VehicleControl/Data Inport/SDFA-L3/Subsystem90 ==
  BusCreator : BusCreator  Inputs=10
  Data Type Conversion{1..3,92} (4 alike) : DataTypeConversion  OutDataTypeStr=single
  Ground{,1..5} (6 alike) : Ground
  Read CM Dict1 : CarMaker4SL/Read CM Dict  xname=User.IO.Out.XAcceleration_S0_002  xsync=off
  Read CM Dict2 : CarMaker4SL/Read CM Dict  xname=User.IO.Out.XAcceleration_S0_003  xsync=off
  Read CM Dict3 : CarMaker4SL/Read CM Dict  xname=User.IO.Out.XAcceleration_S0_004  xsync=off
  Read CM Dict5 : CarMaker4SL/Read CM Dict  xname=User.IO.Out.XAcceleration_S0_001  xsync=off
  LBtar_Xacceleration : Outport
  wires:
  Data Type Conversion92/1 -> BusCreator/1
  Data Type Conversion2/1 -> BusCreator/3
  Data Type Conversion3/1 -> BusCreator/4
  Data Type Conversion1/1 -> BusCreator/2
  BusCreator/1 -> LBtar_Xacceleration/1
  Read CM Dict3/1 -> Data Type Conversion3/1
  Read CM Dict2/1 -> Data Type Conversion2/1
  Read CM Dict1/1 -> Data Type Conversion1/1
  Read CM Dict5/1 -> Data Type Conversion92/1
  Ground/1 -> BusCreator/5
  Ground1/1 -> BusCreator/6
  Ground2/1 -> BusCreator/7
  Ground3/1 -> BusCreator/8
  Ground4/1 -> BusCreator/9
  Ground5/1 -> BusCreator/10

== system MIL4L3_SW6_V1_20220211/CarMaker/VehicleControl/Data Inport/SDFA-L3/Subsystem91 ==
  BusCreator : BusCreator  Inputs=10
  Data Type Conversion{1..3,92} (4 alike) : DataTypeConversion  OutDataTypeStr=single
  Ground{,1..5} (6 alike) : Ground
  Read CM Dict1 : CarMaker4SL/Read CM Dict  xname=User.IO.Out.YAcceleration_S0_002  xsync=off
  Read CM Dict2 : CarMaker4SL/Read CM Dict  xname=User.IO.Out.YAcceleration_S0_003  xsync=off
  Read CM Dict3 : CarMaker4SL/Read CM Dict  xname=User.IO.Out.YAcceleration_S0_004  xsync=off
  Read CM Dict5 : CarMaker4SL/Read CM Dict  xname=User.IO.Out.YAcceleration_S0_001  xsync=off
  LBtar_Yacceleration : Outport
  wires:
  Data Type Conversion92/1 -> BusCreator/1
  Data Type Conversion3/1 -> BusCreator/4
  Data Type Conversion2/1 -> BusCreator/3
  Data Type Conversion1/1 -> BusCreator/2
  Ground5/1 -> BusCreator/10
  Ground4/1 -> BusCreator/9
  Ground3/1 -> BusCreator/8
  Ground2/1 -> BusCreator/7
  Ground1/1 -> BusCreator/6
  Ground/1 -> BusCreator/5
  Read CM Dict5/1 -> Data Type Conversion92/1
  Read CM Dict1/1 -> Data Type Conversion1/1
  Read CM Dict2/1 -> Data Type Conversion2/1
  Read CM Dict3/1 -> Data Type Conversion3/1
  BusCreator/1 -> LBtar_Yacceleration/1

== system MIL4L3_SW6_V1_20220211/CarMaker/VehicleControl/Data Inport/SDFA-L3/Subsystem92 ==
  BusCreator : BusCreator  Inputs=10
  Data Type Conversion{1..3,92} (4 alike) : DataTypeConversion  OutDataTypeStr=single
  Ground{,1..5} (6 alike) : Ground
  Read CM Dict1 : CarMaker4SL/Read CM Dict  xname=User.IO.Out.Width_S0_002  xsync=off
  Read CM Dict2 : CarMaker4SL/Read CM Dict  xname=User.IO.Out.Width_S0_003  xsync=off
  Read CM Dict3 : CarMaker4SL/Read CM Dict  xname=User.IO.Out.Width_S0_004  xsync=off
  Read CM Dict5 : CarMaker4SL/Read CM Dict  xname=User.IO.Out.Width_S0_001  xsync=off
  LBtar_Width : Outport
  wires:
  Data Type Conversion92/1 -> BusCreator/1
  Data Type Conversion3/1 -> BusCreator/4
  Data Type Conversion2/1 -> BusCreator/3
  Data Type Conversion1/1 -> BusCreator/2
  BusCreator/1 -> LBtar_Width/1
  Read CM Dict3/1 -> Data Type Conversion3/1
  Read CM Dict2/1 -> Data Type Conversion2/1
  Read CM Dict1/1 -> Data Type Conversion1/1
  Read CM Dict5/1 -> Data Type Conversion92/1
  Ground/1 -> BusCreator/5
  Ground1/1 -> BusCreator/6
  Ground2/1 -> BusCreator/7
  Ground3/1 -> BusCreator/8
  Ground4/1 -> BusCreator/9
  Ground5/1 -> BusCreator/10

== system MIL4L3_SW6_V1_20220211/CarMaker/VehicleControl/Data Inport/SDFA-L3/Subsystem93 ==
  BusCreator : BusCreator  Inputs=10
  Data Type Conversion{1..3,92} (4 alike) : DataTypeConversion  OutDataTypeStr=single
  Ground{,1..5} (6 alike) : Ground
  Read CM Dict1 : CarMaker4SL/Read CM Dict  xname=User.IO.Out.Length_S0_002  xsync=off
  Read CM Dict2 : CarMaker4SL/Read CM Dict  xname=User.IO.Out.Length_S0_003  xsync=off
  Read CM Dict3 : CarMaker4SL/Read CM Dict  xname=User.IO.Out.Length_S0_004  xsync=off
  Read CM Dict5 : CarMaker4SL/Read CM Dict  xname=User.IO.Out.Length_S0_001  xsync=off
  LBtar_Length : Outport
  wires:
  Data Type Conversion92/1 -> BusCreator/1
  Data Type Conversion2/1 -> BusCreator/3
  Data Type Conversion1/1 -> BusCreator/2
  Data Type Conversion3/1 -> BusCreator/4
  Ground5/1 -> BusCreator/10
  Ground4/1 -> BusCreator/9
  Ground3/1 -> BusCreator/8
  Ground2/1 -> BusCreator/7
  Ground1/1 -> BusCreator/6
  Ground/1 -> BusCreator/5
  Read CM Dict5/1 -> Data Type Conversion92/1
  Read CM Dict1/1 -> Data Type Conversion1/1
  Read CM Dict2/1 -> Data Type Conversion2/1
  Read CM Dict3/1 -> Data Type Conversion3/1
  BusCreator/1 -> LBtar_Length/1

== system MIL4L3_SW6_V1_20220211/CarMaker/VehicleControl/Data Inport/SDFA-L3/Subsystem94 ==
  BusCreator : BusCreator  Inputs=10
  Data Type Conversion{1..3,92} (4 alike) : DataTypeConversion  OutDataTypeStr=single
  Ground{,1..5} (6 alike) : Ground
  Read CM Dict1 : CarMaker4SL/Read CM Dict  xname=User.IO.Out.Orientation_S0_002  xsync=off
  Read CM Dict2 : CarMaker4SL/Read CM Dict  xname=User.IO.Out.Orientation_S0_003  xsync=off
  Read CM Dict3 : CarMaker4SL/Read CM Dict  xname=User.IO.Out.Orientation_S0_004  xsync=off
  Read CM Dict5 : CarMaker4SL/Read CM Dict  xname=User.IO.Out.Orientation_S0_001  xsync=off
  LBtar_Orientation : Outport
  wires:
  Data Type Conversion92/1 -> BusCreator/1
  Data Type Conversion1/1 -> BusCreator/2
  Data Type Conversion3/1 -> BusCreator/4
  Data Type Conversion2/1 -> BusCreator/3
  BusCreator/1 -> LBtar_Orientation/1
  Read CM Dict3/1 -> Data Type Conversion3/1
  Read CM Dict2/1 -> Data Type Conversion2/1
  Read CM Dict1/1 -> Data Type Conversion1/1
  Read CM Dict5/1 -> Data Type Conversion92/1
  Ground/1 -> BusCreator/5
  Ground1/1 -> BusCreator/6
  Ground2/1 -> BusCreator/7
  Ground3/1 -> BusCreator/8
  Ground4/1 -> BusCreator/9
  Ground5/1 -> BusCreator/10

== system MIL4L3_SW6_V1_20220211/CarMaker/VehicleControl/Data Inport/SDFA-L3/Subsystem95 ==
  BusCreator : BusCreator  Inputs=10
  Data Type Conversion{1..3,92} (4 alike) : DataTypeConversion  OutDataTypeStr=single
  Ground{,1..5} (6 alike) : Ground
  Read CM Dict1 : CarMaker4SL/Read CM Dict  xname=User.IO.Out.ExistenceProbability_S0_002  xsync=off
  Read CM Dict2 : CarMaker4SL/Read CM Dict  xname=User.IO.Out.ExistenceProbability_S0_003  xsync=off
  Read CM Dict3 : CarMaker4SL/Read CM Dict  xname=User.IO.Out.ExistenceProbability_S0_004  xsync=off
  Read CM Dict5 : CarMaker4SL/Read CM Dict  xname=User.IO.Out.ExistenceProbability_S0_001  xsync=off
  LBtar_ExistenceProbability : Outport
  wires:
  Data Type Conversion92/1 -> BusCreator/1
  Data Type Conversion2/1 -> BusCreator/3
  Data Type Conversion3/1 -> BusCreator/4
  Data Type Conversion1/1 -> BusCreator/2
  Ground5/1 -> BusCreator/10
  Ground4/1 -> BusCreator/9
  Ground3/1 -> BusCreator/8
  Ground2/1 -> BusCreator/7
  Ground1/1 -> BusCreator/6
  Ground/1 -> BusCreator/5
  Read CM Dict5/1 -> Data Type Conversion92/1
  Read CM Dict1/1 -> Data Type Conversion1/1
  Read CM Dict2/1 -> Data Type Conversion2/1
  Read CM Dict3/1 -> Data Type Conversion3/1
  BusCreator/1 -> LBtar_ExistenceProbability/1

== system MIL4L3_SW6_V1_20220211/CarMaker/VehicleControl/Data Inport/SDFA-L3/Subsystem96 ==
  BusCreator : BusCreator  Inputs=10
  Data Type Conversion{1..3,144} (4 alike) : DataTypeConversion  OutDataTypeStr=uint8
  Ground{,1..5} (6 alike) : Ground
  Read CM Dict1 : CarMaker4SL/Read CM Dict  xname=User.IO.Out.ClassHighest_S0_002  xsync=off
  Read CM Dict2 : CarMaker4SL/Read CM Dict  xname=User.IO.Out.ClassHighest_S0_003  xsync=off
  Read CM Dict3 : CarMaker4SL/Read CM Dict  xname=User.IO.Out.ClassHighest_S0_004  xsync=off
  Read CM Dict5 : CarMaker4SL/Read CM Dict  xname=User.IO.Out.ClassHighest_S0_001  xsync=off
  LBtar_Class : Outport
  wires:
  Data Type Conversion3/1 -> BusCreator/4
  Data Type Conversion2/1 -> BusCreator/3
  Data Type Conversion1/1 -> BusCreator/2
  Data Type Conversion144/1 -> BusCreator/1
  BusCreator/1 -> LBtar_Class/1
  Read CM Dict3/1 -> Data Type Conversion3/1
  Read CM Dict2/1 -> Data Type Conversion2/1
  Read CM Dict1/1 -> Data Type Conversion1/1
  Read CM Dict5/1 -> Data Type Conversion144/1
  Ground/1 -> BusCreator/5
  Ground1/1 -> BusCreator/6
  Ground2/1 -> BusCreator/7
  Ground3/1 -> BusCreator/8
  Ground4/1 -> BusCreator/9
  Ground5/1 -> BusCreator/10

== system MIL4L3_SW6_V1_20220211/CarMaker/VehicleControl/Data Inport/SDFA-L3/Subsystem97 ==
  BusCreator : BusCreator  Inputs=10
  Data Type Conversion{1..3,92} (4 alike) : DataTypeConversion  OutDataTypeStr=single
  Ground{,1..5} (6 alike) : Ground
  Read CM Dict1 : CarMaker4SL/Read CM Dict  xname=User.IO.Out.ReferencePoint_S0_002  xsync=off
  Read CM Dict2 : CarMaker4SL/Read CM Dict  xname=User.IO.Out.ReferencePoint_S0_003  xsync=off
  Read CM Dict3 : CarMaker4SL/Read CM Dict  xname=User.IO.Out.ReferencePoint_S0_004  xsync=off
  Read CM Dict5 : CarMaker4SL/Read CM Dict  xname=User.IO.Out.ReferencePoint_S0_001  xsync=off
  LBtar_ReferencePoint : Outport
  wires:
  Data Type Conversion3/1 -> BusCreator/4
  Data Type Conversion2/1 -> BusCreator/3
  Data Type Conversion92/1 -> BusCreator/1
  Data Type Conversion1/1 -> BusCreator/2
  Ground5/1 -> BusCreator/10
  Ground4/1 -> BusCreator/9
  Ground3/1 -> BusCreator/8
  Ground2/1 -> BusCreator/7
  Ground1/1 -> BusCreator/6
  Ground/1 -> BusCreator/5
  Read CM Dict5/1 -> Data Type Conversion92/1
  Read CM Dict1/1 -> Data Type Conversion1/1
  Read CM Dict2/1 -> Data Type Conversion2/1
  Read CM Dict3/1 -> Data Type Conversion3/1
  BusCreator/1 -> LBtar_ReferencePoint/1

== system MIL4L3_SW6_V1_20220211/CarMaker/VehicleControl/Data Inport/SDFA-L3/Subsystem98 ==
  BusCreator : BusCreator  Inputs=10
  Data Type Conversion{1..3,92} (4 alike) : DataTypeConversion  OutDataTypeStr=single
  Ground{,1..5} (6 alike) : Ground
  Read CM Dict1 : CarMaker4SL/Read CM Dict  xname=User.IO.Out.MovingState_S0_002  xsync=off
  Read CM Dict2 : CarMaker4SL/Read CM Dict  xname=User.IO.Out.MovingState_S0_003  xsync=off
  Read CM Dict3 : CarMaker4SL/Read CM Dict  xname=User.IO.Out.MovingState_S0_004  xsync=off
  Read CM Dict5 : CarMaker4SL/Read CM Dict  xname=User.IO.Out.MovingState_S0_001  xsync=off
  LBtar_MovingState : Outport
  wires:
  Data Type Conversion92/1 -> BusCreator/1
  Data Type Conversion2/1 -> BusCreator/3
  Data Type Conversion3/1 -> BusCreator/4
  Data Type Conversion1/1 -> BusCreator/2
  BusCreator/1 -> LBtar_MovingState/1
  Read CM Dict3/1 -> Data Type Conversion3/1
  Read CM Dict2/1 -> Data Type Conversion2/1
  Read CM Dict1/1 -> Data Type Conversion1/1
  Read CM Dict5/1 -> Data Type Conversion92/1
  Ground/1 -> BusCreator/5
  Ground1/1 -> BusCreator/6
  Ground2/1 -> BusCreator/7
  Ground3/1 -> BusCreator/8
  Ground4/1 -> BusCreator/9
  Ground5/1 -> BusCreator/10

== system MIL4L3_SW6_V1_20220211/CarMaker/VehicleControl/Function/ICA/EPS Position Control Enable Management (EPSPCEM)_KDK1 ==
  EPSPCEM__bsTHState : Inport
  EPS_Ctr_State : Inport  Port=2
  Data Type Conversion : DataTypeConversion  OutDataTypeStr=uint16
  EPS_Ctr_Disable : Subsystem  TreatAsAtomicUnit=on
  EPS_Ctr_Enable : Subsystem  TreatAsAtomicUnit=on
  If1 : If  IfExpression=u1 ~= 0
  Merge1 : Merge
  stEPS_State_Ctl_CMD : Outport
  wires:
  EPS_Ctr_Disable/1(stEPSCtlCMD) -> Merge1/2
  If1/2 -> EPS_Ctr_Disable/Action
  EPS_Ctr_State/1 -> EPS_Ctr_Disable/1(stEPSCtlState), EPS_Ctr_Enable/1(stEPSCtlState)
  EPSPCEM__bsTHState/1 -> If1/1
  EPS_Ctr_Enable/1(stEPSCtlCMD) -> Merge1/1
  Merge1/1 -> Data Type Conversion/1
  If1/1 -> EPS_Ctr_Enable/Action
  Data Type Conversion/1 -> stEPS_State_Ctl_CMD/1

== system MIL4L3_SW6_V1_20220211/CarMaker/VehicleControl/Function/ICA/EPS_State_Mashine ==
  EPS_CMD_KDK : Inport
  Data Type Conversion : DataTypeConversion  OutDataTypeStr=uint16
  Data Type Conversion1 : DataTypeConversion  OutDataTypeStr=uint16
  EPS_Default : Constant  Value=0
  EPS_Other_Con : Constant
  Steering Angle Cmd Synthesis State Machine (SWASynSM) : Stateflow chart  TreatAsAtomicUnit=on
  EPS_Ctr_State : Outport
  wires:
  EPS_CMD_KDK/1 -> Steering Angle Cmd Synthesis State Machine (SWASynSM)/1(EPS_CMD_KDK)
  EPS_Other_Con/1 -> Data Type Conversion/1
  EPS_Default/1 -> Data Type Conversion1/1
  Data Type Conversion/1 -> Steering Angle Cmd Synthesis State Machine (SWASynSM)/2(EPS_Other_Con)
  Data Type Conversion1/1 -> Steering Angle Cmd Synthesis State Machine (SWASynSM)/3(EPS_Default)
  Steering Angle Cmd Synthesis State Machine (SWASynSM)/1(EPS_Ctr_State) -> EPS_Ctr_State/1

== system MIL4L3_SW6_V1_20220211/CarMaker/VehicleControl/Function/ICA/Enabled Subsystem ==
  In : Inport
  Enable : EnablePort
  Compare To Constant : simulink/Logic and Bit Operations/Compare To Constant  relop===  const=4  OutDataTypeStr=boolean
  Out1 : Outport
  wires:
  In/1 -> Compare To Constant/1
  Compare To Constant/1 -> Out1/1

== system MIL4L3_SW6_V1_20220211/CarMaker/VehicleControl/Function/ICA_ALC/EPS Position Control Enable Management (EPSPCEM)_KDK1 ==
  note: eps_lka_state
  note: ica_mode
  EPSPCEM__bsTHmode : Inport
  EPS_Ctr_State : Inport  Port=2
  Data Type Conversion : DataTypeConversion  OutDataTypeStr=uint16
  EPS_Ctr_Disable : Subsystem  TreatAsAtomicUnit=on
  EPS_Ctr_Enable : Subsystem  TreatAsAtomicUnit=on
  If1 : If  IfExpression=u1 ~= 0
  Merge1 : Merge
  stEPS_State_Ctl_CMD : Outport
  wires:
  Data Type Conversion/1 -> stEPS_State_Ctl_CMD/1
  If1/1 -> EPS_Ctr_Enable/Action
  Merge1/1 -> Data Type Conversion/1
  EPS_Ctr_Enable/1(stEPSCtlCMD) -> Merge1/1
  EPSPCEM__bsTHmode/1 -> If1/1
  EPS_Ctr_State/1 -> EPS_Ctr_Enable/1(stEPSCtlState), EPS_Ctr_Disable/1(stEPSCtlState)
  If1/2 -> EPS_Ctr_Disable/Action
  EPS_Ctr_Disable/1(stEPSCtlCMD) -> Merge1/2

== system MIL4L3_SW6_V1_20220211/CarMaker/VehicleControl/Function/ICA_ALC/EPS_State_Mashine ==
  EPS_CMD_KDK : Inport
  Data Type Conversion : DataTypeConversion  OutDataTypeStr=uint16
  Data Type Conversion1 : DataTypeConversion  OutDataTypeStr=uint16
  EPS_Default : Constant  Value=0
  EPS_Other_Con : Constant
  Steering Angle Cmd Synthesis State Machine (SWASynSM) : Stateflow chart  TreatAsAtomicUnit=on
  EPS_Ctr_State : Outport
  wires:
  Steering Angle Cmd Synthesis State Machine (SWASynSM)/1(EPS_Ctr_State) -> EPS_Ctr_State/1
  Data Type Conversion1/1 -> Steering Angle Cmd Synthesis State Machine (SWASynSM)/3(EPS_Default)
  Data Type Conversion/1 -> Steering Angle Cmd Synthesis State Machine (SWASynSM)/2(EPS_Other_Con)
  EPS_Default/1 -> Data Type Conversion1/1
  EPS_Other_Con/1 -> Data Type Conversion/1
  EPS_CMD_KDK/1 -> Steering Angle Cmd Synthesis State Machine (SWASynSM)/1(EPS_CMD_KDK)

== system MIL4L3_SW6_V1_20220211/CarMaker/VehicleControl/Function/ICA_ALC/Enabled Subsystem ==
  In : Inport
  Enable : EnablePort
  Compare To Constant : simulink/Logic and Bit Operations/Compare To Constant  relop===  const=4  OutDataTypeStr=boolean
  Out1 : Outport
  wires:
  Compare To Constant/1 -> Out1/1
  In/1 -> Compare To Constant/1
